simulink library "atmModelLib"  (R2021b)
settings: Solver=VariableStepAuto  StartTime=0.0  StopTime=10.0  RelTol=1e-3
undefined symbols (not defined in the file): atmModel
settings Model: Creator=mat  LastModifiedBy=mat

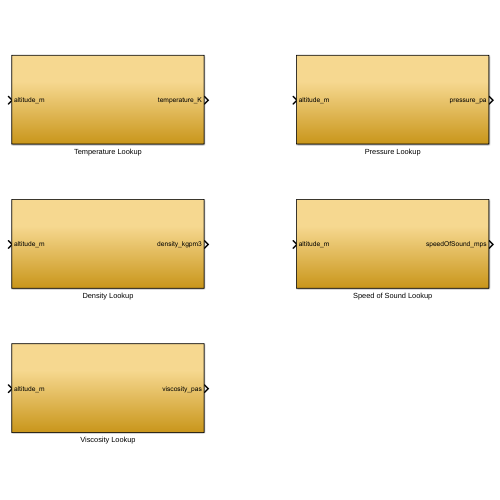
[thumbnail: Simulink's stored preview of the top-level diagram]
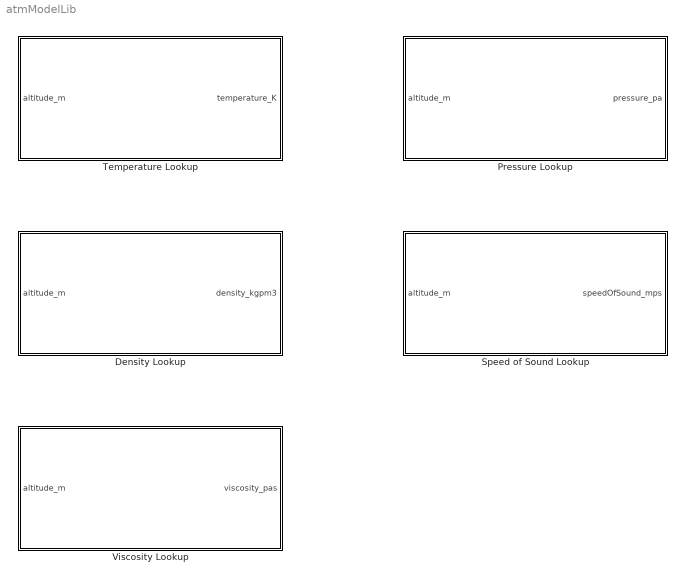
== system atmModelLib ==
  Density Lookup : Subsystem
  Pressure Lookup : Subsystem
  Speed of Sound Lookup : Subsystem
  Temperature Lookup : Subsystem
  Viscosity Lookup : Subsystem

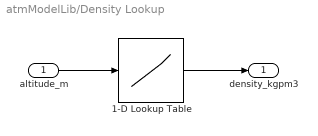
== system atmModelLib/Density Lookup ==
  altitude_m : Inport
  1-D Lookup Table : Lookup_n-D  NumberOfTableDimensions=1  BreakpointsForDimension1=atmModel.altitudeBreakpoints_m  Table=atmModel.density_kgpm3  InternalRulePriority=Speed  RndMeth=Simplest  InputSameDT=on
  density_kgpm3 : Outport
  wires:
  altitude_m/1 -> 1-D Lookup Table/1
  1-D Lookup Table/1 -> density_kgpm3/1

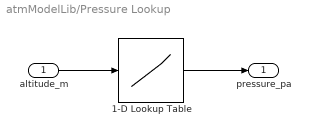
== system atmModelLib/Pressure Lookup ==
  altitude_m : Inport
  1-D Lookup Table : Lookup_n-D  NumberOfTableDimensions=1  BreakpointsForDimension1=atmModel.altitudeBreakpoints_m  Table=atmModel.pressure_pa  InternalRulePriority=Speed  RndMeth=Simplest  InputSameDT=on
  pressure_pa : Outport
  wires:
  1-D Lookup Table/1 -> pressure_pa/1
  altitude_m/1 -> 1-D Lookup Table/1

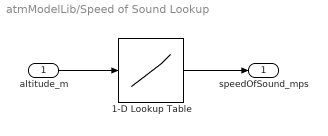
== system atmModelLib/Speed of Sound Lookup ==
  altitude_m : Inport
  1-D Lookup Table : Lookup_n-D  NumberOfTableDimensions=1  BreakpointsForDimension1=atmModel.altitudeBreakpoints_m  Table=atmModel.speedOfSound_mps  InternalRulePriority=Speed  RndMeth=Simplest  InputSameDT=on
  speedOfSound_mps : Outport
  wires:
  1-D Lookup Table/1 -> speedOfSound_mps/1
  altitude_m/1 -> 1-D Lookup Table/1

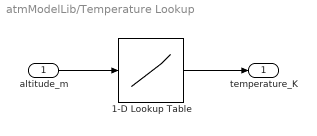
== system atmModelLib/Temperature Lookup ==
  altitude_m : Inport
  1-D Lookup Table : Lookup_n-D  NumberOfTableDimensions=1  BreakpointsForDimension1=atmModel.altitudeBreakpoints_m  Table=atmModel.temperature_K  InternalRulePriority=Speed  RndMeth=Simplest  InputSameDT=on
  temperature_K : Outport
  wires:
  altitude_m/1 -> 1-D Lookup Table/1
  1-D Lookup Table/1 -> temperature_K/1

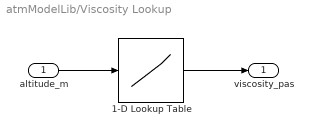
== system atmModelLib/Viscosity Lookup ==
  altitude_m : Inport
  1-D Lookup Table : Lookup_n-D  NumberOfTableDimensions=1  BreakpointsForDimension1=atmModel.altitudeBreakpoints_m  Table=atmModel.viscosity_pas  InternalRulePriority=Speed  RndMeth=Simplest  InputSameDT=on
  viscosity_pas : Outport
  wires:
  altitude_m/1 -> 1-D Lookup Table/1
  1-D Lookup Table/1 -> viscosity_pas/1
